simulink model "FLIGHT_hexacopter"  (R2024a)
settings: Solver=FixedStepDiscrete  StartTime=0.0  StopTime=inf  FixedStep=SampleTime_SAS  RelTol=1e-3  EnableMultiTasking=on
InitFcn:
  | Init_FLIGHT_Hexacopter
values from neighbouring files (symbols this model uses):
  d2r = pi/180    (= 0.0174532925199)    [Init_FLIGHT_Hexacopter.m]
  Kdpr = 0.004    [Init_FLIGHT_Hexacopter_fromNCMS.m]
  Kdrr = 0.004    [Init_FLIGHT_Hexacopter_fromNCMS.m]
  Kdvz = 0.0254    [Init_FLIGHT_Hexacopter_fromNCMS.m]
  Kdyr = 0.0298    [Init_FLIGHT_Hexacopter_fromNCMS.m]
  Kipr = 0.0    (= 0)    [Init_FLIGHT_Hexacopter_fromNCMS.m]
  Kirr = 0.0    (= 0)    [Init_FLIGHT_Hexacopter_fromNCMS.m]
  Kivz = 0.6304    [Init_FLIGHT_Hexacopter_fromNCMS.m]
  Kiyr = 0.0    (= 0)    [Init_FLIGHT_Hexacopter_fromNCMS.m]
  Kpp = 3.3894    [Init_FLIGHT_Hexacopter_fromNCMS.m]
  Kppr = 0.1    [Init_FLIGHT_Hexacopter_fromNCMS.m]
  Kpr = 3.3894    [Init_FLIGHT_Hexacopter_fromNCMS.m]
  Kprr = 0.1    [Init_FLIGHT_Hexacopter_fromNCMS.m]
  Kpvz = 0.3191    [Init_FLIGHT_Hexacopter_fromNCMS.m]
  Kpyr = 0.3744    [Init_FLIGHT_Hexacopter_fromNCMS.m]
  MAX_CONTROL_ANGLE_PITCH = 30*pi/180    (= 0.523598775598)    [Init_FLIGHT_Hexacopter.m]    (also in Init_FLIGHT_Hexacopter_fromNCMS.m = 0.349065850399)
  MAX_CONTROL_ANGLE_RATE_PITCH = 360*pi/180    (= 6.28318530718)    [Init_FLIGHT_Hexacopter.m]    (also in Init_FLIGHT_Hexacopter_fromNCMS.m)
  MAX_CONTROL_ANGLE_RATE_ROLL = 360*pi/180    (= 6.28318530718)    [Init_FLIGHT_Hexacopter.m]    (also in Init_FLIGHT_Hexacopter_fromNCMS.m)
  MAX_CONTROL_ANGLE_RATE_Y = 120*pi/180    (= 2.09439510239)    [Init_FLIGHT_Hexacopter.m]    (also in Init_FLIGHT_Hexacopter_fromNCMS.m)
  MAX_CONTROL_ANGLE_ROLL = 30*pi/180    (= 0.523598775598)    [Init_FLIGHT_Hexacopter.m]    (also in Init_FLIGHT_Hexacopter_fromNCMS.m = 0.349065850399)
  MAX_CONTROL_VELOCITY_XY = 1.5    [Init_FLIGHT_Hexacopter.m]    (also in Init_FLIGHT_Hexacopter_fromNCMS.m)
  MAX_CONTROL_VELOCITY_Z = 1    [Init_FLIGHT_Hexacopter.m]    (also in Init_FLIGHT_Hexacopter_fromNCMS.m)
  Npr = 50    [Init_FLIGHT_Hexacopter_fromNCMS.m]
  Nrr = 50    [Init_FLIGHT_Hexacopter_fromNCMS.m]
  Nvz = Npr    (= 50)    [Init_FLIGHT_Hexacopter_fromNCMS.m]
  Nyr = 50    [Init_FLIGHT_Hexacopter_fromNCMS.m]
  SampleTime = 1/200    (= 0.005)    [Init_FLIGHT_Hexacopter.m]    (also in Init_FLIGHT_Hexacopter_fromNCMS.m = 0.01)
  SampleTime_SAS = 1/1000    (= 0.001)    [Init_FLIGHT_Hexacopter.m]
undefined symbols (not defined in the file or in its folder): arguments, event_sequence, id, log_levels, MPC_Z_D, MPC_Z_I, MPC_Z_P, noutputs, output, pitch, pitch_body, q_d, roll, roll_body, thrust_body, timestamp, vx, vy, vz, x, y, yaw, yaw_sp_move_rate, z
libraries: px4lib x35, px4uORBlib x12, px4Utilslib x11, slpidlib x10, simulink x3, simulink_extras x2, px4Sensorslib x2, sharedtransform x1
(part 3 of 3)

== system FLIGHT_hexacopter/If Action Subsystem/XY Velocity Controller ==
  des_vxvy : Inport
  vxvy : Inport  Port=2
  Pos : Inport  Port=3
  Enable : EnablePort
  Demux : Demux  Outputs=2
  Gain1 : Gain  Gain=-1
  NED2Body1 : Subsystem
  PID_Altitude : slpidlib/PID Controller  Controller=P  Form=Parallel  TimeDomain=Discrete-time  UseExternalTs=off  SampleTime=-1  IntegratorMethod=Backward Euler  FilterMethod=Forward Euler  ControllerParametersSource=external  P=MPC_Z_P  I=MPC_Z_I  UseKiTs=off  D=MPC_Z_D  UseExternalDerivativeSource=off  N=10  UseFilter=on  TunerSelectOption=Transfer Function Based (PID Tuner App)  InitialConditionSource=internal  InitialConditionForIntegrator=0  InitialConditionForFilter=0  DifferentiatorICPrevScaledInput=0  ExternalReset=none  TrackingMode=off  Kt=1  LimitOutput=off  SatLimitsSource=internal  UpperSaturationLimit=inf  LowerSaturationLimit=-inf  LinearizeAsGain=off  AntiWindupMode=clamping  Kb=1  LimitIntegrator=off  UpperIntegratorSaturationLimit=inf  LowerIntegratorSaturationLimit=-inf  POutMin=[]  POutMax=[]  IOutMin=[]  IOutMax=[]  DOutMin=[]  DOutMax=[]  NOutMin=[]  NOutMax=[]  SumOutMin=[]  SumOutMax=[]  SaturationOutMin=[]  SaturationOutMax=[]  PParamMin=[]  PParamMax=[]  IParamMin=[]  IParamMax=[]  DParamMin=[]  DParamMax=[]  NParamMin=[]  NParamMax=[]  KbParamMin=[]  KbParamMax=[]  KtParamMin=[]  KtParamMax=[]  KbOutMin=[]  KbOutMax=[]  KtOutMin=[]  KtOutMax=[]  IntegratorOutMin=[]  IntegratorOutMax=[]  FilterOutMin=[]  FilterOutMax=[]  SumI1OutMin=[]  SumI1OutMax=[]  SumI2OutMin=[]  SumI2OutMax=[]  SumI3OutMin=[]  SumI3OutMax=[]  SumI4OutMin=[]  SumI4OutMax=[]  SumDOutMin=[]  SumDOutMax=[]  DifferentiatorOutMin=[]  DifferentiatorOutMax=[]  FilterDiffOutCoefMin=[]  FilterDiffOutCoefMax=[]  ReciprocalOutMin=[]  ReciprocalOutMax=[]  SumDenOutMin=[]  SumDenOutMax=[]  SumNumOutMin=[]  SumNumOutMax=[]  DivideOutMin=[]  DivideOutMax=[]  UdiffTsProdOutMin=[]  UdiffTsProdOutMax=[]  NTsProdOutMin=[]  NTsProdOutMax=[]  UintegralTsProdOutMin=[]  UintegralTsProdOutMax=[]  UngainTsProdOutMin=[]  UngainTsProdOutMax=[]  ClampingZeroOutDataTypeStr=Inherit: Inherit via back propagation  ClampingZeroOutMin=[]  ClampingZeroOutMax=[]  FilterDenConstantOutDataTypeStr=Inherit: Inherit via back propagation  FilterDenConstantOutMin=[]  FilterDenConstantOutMax=[]  PCopyOutDataTypeStr=Inherit: Inherit via back propagation  PCopyOutMin=[]  PCopyOutMax=[]  NCopyOutDataTypeStr=Inherit: Inherit via back propagation  NCopyOutMin=[]  NCopyOutMax=[]  IntegratorContinuousStateAttributes=''  IntegratorStateMustResolveToSignalObject=off  IntegratorRTWStateStorageClass=Auto  FilterContinuousStateAttributes=''  FilterStateMustResolveToSignalObject=off  FilterRTWStateStorageClass=Auto  ParallelPVariant=ExternalParameters  IdealPVariant=Disabled  IVariant=Disabled  DVariant=Disabled  IntegratorVariant=Disabled  SatVariant=Disabled  AWVariant=Disabled  PCopyVariant=Disabled  TRVariant=Disabled  FdbkBlocksVariant=Forward  IdealPFdbkVariant=Disabled  SatFdbkVariant=Disabled  DerivativeFilterVariant=Disabled  NVariant=Disabled  NCopyVariant=Disabled_SignalSpec  FilterICVariant=Disabled  IntegratorICVariant=Disabled  ExternalResetVariant=Disabled  TRSumVariant=Passthrough  SumFdbkVariant=Disabled  SumVariant=Passthrough_P  TsampFilterVariant=InternalTs  TsampNgainVariant=Passthrough  TsampIntegralVariant=Disabled_SignalSpec  ExternalSaturationOutDataTypeStr=Inherit: Same as second input  DerivativeSourceVariant=Disabled
  Read Parameter : px4lib/Read Parameter  ParameterName=MPC_XY_VEL_P_ACC  DataType=FLOAT  SampleTime=SampleTime
      settings: SourceProductName=UAV Toolbox Support Package for PX4 Autopilots
  Saturation : Saturate  UpperLimit=35*d2r  LowerLimit=-35*d2r
  Selector : Selector  InputPortWidth=4  IndexOptions=Index vector (dialog)  Indices=4  OutputSizes=1
  Sum : Sum  Inputs=|+-
  Terminator : Terminator
  des_pitch : Outport
  des_roll : Outport  Port=2
  wires:
  Demux/1 -> Gain1/1
  Demux/2 -> des_roll/1
  Gain1/1 -> des_pitch/1
  PID_Altitude/1 -> Saturation/1  "vz_cmd"
  Saturation/1 -> Demux/1
  Pos/1 -> Selector/1
  [heading] -> NED2Body1/2(Heading)
  des_vxvy/1 -> Sum/1
  Selector/1 -> [heading]
  vxvy/1 -> Sum/2
  Sum/1 -> NED2Body1/1(NED)
  NED2Body1/1(BODY) -> PID_Altitude/1
  Read Parameter/2 -> Terminator/1
  Read Parameter/1 -> PID_Altitude/2

== system FLIGHT_hexacopter/Remote Control/Arm1 ==
  Arm : Inport
  Compare To Constant3 : simulink/Logic and Bit Operations/Compare To Constant  relop=>=  const=uint16(1800)  OutDataTypeStr=boolean
  Arm_cmd : Outport  VectorParamsAs1DForOutWhenUnconnected=off
  wires:
  Arm/1 -> Compare To Constant3/1
  Compare To Constant3/1 -> Arm_cmd/1

== system FLIGHT_hexacopter/actuator_outputs_motors/Normalize_pwm6 ==
  In1 : Inport
  Constant : Constant  Value=1000  OutDataTypeStr=single  SampleTime=SampleTime_SAS
  Gain : Gain  Gain=1/1000
  Saturation : Saturate  UpperLimit=2000  LowerLimit=1000
  Subtract : Sum  Inputs=+-
  Out1 : Outport
  wires:
  In1/1 -> Saturation/1
  Saturation/1 -> Subtract/1
  Constant/1 -> Subtract/2
  Subtract/1 -> Gain/1
  Gain/1 -> Out1/1

== system FLIGHT_hexacopter/uORB_actuator_outputs1/Normalize_pwm6 ==
  In1 : Inport
  Constant : Constant  Value=1000  OutDataTypeStr=single
  Gain : Gain  Gain=1/1000
  Saturation : Saturate  UpperLimit=2000  LowerLimit=1000
  Subtract : Sum  Inputs=+-
  Out1 : Outport
  wires:
  In1/1 -> Saturation/1
  Saturation/1 -> Subtract/1
  Constant/1 -> Subtract/2
  Subtract/1 -> Gain/1
  Gain/1 -> Out1/1

== system FLIGHT_hexacopter/If Action Subsystem/XY Velocity Controller/NED2Body1 ==
  NED : Inport
  Heading : Inport  Port=2
  Calculate Transformation Matrix : Subsystem
  MatrixMultiply : Product  Multiplication=Matrix(*)
  BODY : Outport
  wires:
  Calculate Transformation Matrix/1(R) -> MatrixMultiply/1
  Heading/1 -> Calculate Transformation Matrix/1(theta)
  NED/1 -> MatrixMultiply/2
  MatrixMultiply/1 -> BODY/1

== system FLIGHT_hexacopter/If Action Subsystem/XY Velocity Controller/NED2Body1/Calculate Transformation Matrix ==
  theta : Inport
  Gain : Gain  Gain=-1
  Matrix Concatenate : Concatenate  Mode=Multidimensional array
  Mux : Mux  Inputs=2
  Mux1 : Mux  Inputs=2
  Reshape : Reshape  OutputDimensionality=Row vector (2-D)
  Reshape1 : Reshape  OutputDimensionality=Row vector (2-D)
  SinCos : Trigonometry  Operator=sincos
  Transpose : Math  Operator=transpose
  R : Outport
  wires:
  Reshape1/1 -> Matrix Concatenate/2
  Reshape/1 -> Matrix Concatenate/1
  Transpose/1 -> R/1
  Matrix Concatenate/1 -> Transpose/1
  Mux1/1 -> Reshape1/1
  Mux/1 -> Reshape/1
  Gain/1 -> Mux/2
  SinCos/1 -> Mux1/1, Gain/1
  SinCos/2 -> Mux/1, Mux1/2
  theta/1 -> SinCos/1

== matlab function FLIGHT_hexacopter/Doublet_Generator/MATLAB Function ==
  data: in_roll input double; in_pitch input double; in_yawrate input double; flag input boolean; out_roll output double; out_pitch output double; out_yawrate output double; time_usec input double; peak_angle_deg input double; doublet_dt input double; doublet_axis input int32
function [out_roll, out_pitch,out_yawrate]= DoubletGenerator(in_roll, in_pitch, in_yawrate, flag, time_usec, peak_angle_deg, doublet_dt, doublet_axis)
persistent start_time_usec;
if(isempty(start_time_usec))
    start_time_usec = -1;
end

if(flag && start_time_usec == -1)
    start_time_usec = time_usec;
end
d2r = pi/180;

if (flag && start_time_usec > 0) % time calculation
    reletive_time_sec = double(time_usec - start_time_usec)*1e-6;
else
    start_time_usec = -1;
    reletive_time_sec = 0;
end

% Define Doublet
t1 = 0;
t2 = t1+doublet_dt;
t3 = t2+doublet_dt;
peak_angle_rad = peak_angle_deg * d2r;

% Default Output
out_roll = in_roll;
out_pitch = in_pitch;
out_yawrate = in_yawrate;

% Generate Doublet Command
if(flag)
    if(reletive_time_sec >= t1 && reletive_time_sec < t2)
        cmd = peak_angle_rad;
    elseif(reletive_time_sec >= t2 && reletive_time_sec < t3)
        cmd = -peak_angle_rad;
    else
        cmd = 0;
    end

    switch(double(doublet_axis))
        case 1
            out_roll = cmd;
        case 2
            out_pitch = cmd;
        case 3
            out_yawrate = cmd;
    end
end

== matlab function FLIGHT_hexacopter/quat2eul ==
  data: q input; ypr output
function ypr  = quat2eul(q)

% Quaternion conversion to Euler angles based on the PX4 Firmware v1.10.2
% release.

phi = atan2(2*(q(1)*q(2) + q(3)* q(4)), q(1)^2 - q(2)^2 - q(3)^2 + q(4)^2);
theta = asin(-2*(q(2)*q(4) - q(1)*q(3)));
psi = atan2(2*(q(2)*q(3) + q(1)* q(4)), q(1)^2 + q(2)^2 - q(3)^2 - q(4)^2);

ypr = [psi theta phi];

end

== matlab function FLIGHT_hexacopter/QP_Allocation/MATLAB Function ==
  data: normalized_thrust_setpoint output size=[1 6]; f_total input; thrust_setpoints output; tau_phi input; tau_theta input; tau_psi input; A input; u_prev input double; failure_status input
function [normalized_thrust_setpoint, thrust_setpoints] = QPBasedControlAllocation(f_total, tau_phi, tau_theta, tau_psi, A, u_prev, failure_status)


% f_total: 추력 명령 [N], tau_phi, tau_theta, tau_psi: 롤 피치 요 토크 명령 [N.m]
% thrust_setpoints: 각 모터별 추력 명령[N] normalized_thrust_setpoint: 모터 최대 출력으로
% 정규화한 값
% A : Control Effectiviness MAtrix
num_actuator = 6;
u_des = [f_total; tau_phi; tau_theta; tau_psi];

% 각 추진기의 추력 제한 정의 (예시 값)
f_min = 0;           % 최소 추력 (뉴턴)
f_max = 7;           % 최대 추력 (뉴턴)

% 목적 함수의 이차 및 선형 계수 정의
% 목적: f' * f (추력의 제곱합 최소화)
H = 2 * eye(num_actuator);      % MATLAB의 quadprog은 (1/2)x'Hx + f'x를 최소화
f_obj = zeros(num_actuator,1);  % 선형 항 없음
%%
scenario = 3; 
numMotors = 6;
switch scenario
    case 1
        % 에너지 최소화: min u'u
        H = eye(numMotors);
        f_obj = zeros(numMotors,1); 
        
    case 2
        % 특정 모터 사용 억제: 모터 #1 가중치↑
        % H = diag([가중치,1,1,1,1,1])
        H = diag([1, 1, 1, 1, 1, 1]);
        f = zeros(numMotors,1);
        
    case 3
        % 추력 변화율 최소화: min (u - u_prev)'(u - u_prev)
        % = u'u - 2 u_prev'u + const
        % quadprog 형식: (1/2)*u'Hu + f'u -> 여기서 H = 2 * I, f = -2 * u_prev로 하면되지만
        % (1/2)을 빼려면 H=I로 하고 f=-2*u_prev을 그대로 써도 동일한 해를 얻기 위해,
        % 여기서는 H=I, f = -2*u_prev로 간단히 처리하겠습니다.
        
        % 실제 quadprog는 (1/2)*H*u'u + f'u를 최소화하므로
        % (1/2)*u'u + (-u_prev')*u = (1/2)*u'u - u_prev'*u
        % 이는 위 식과 상수항 차이만 있고 최소점 동일.
        H = eye(numMotors);
        f_obj = -2*u_prev; 
        % 정확히 하려면 H=2*eye(numMotors), f = -2*u_prev 로 두고,
        % 목적함수를 (1/2)*u'Hu + f'u 형태로 맞출 수 있음.
        % 여기서는 단순화해서 H=I, f=-2*u_prev 사용
        % 이 경우 목적함수는 (1/2)*u'u - u_prev'*u,
        % u'=u-u_prev일 때 상수항 무시하면 동일한 최소점.

        % 좀 더 엄밀히 하려면 다음과 같이 할 수도 있음:
        % H = 2*eye(numMotors);
        % f = -2*u_prev;
        % 이렇게 하면 목적함수는 (1/2)*u'(2I)u + (-2u_prev')u = u'u - u_prev'*u
        % = (u - u_prev)'(u - u_prev) - u_prev'u_prev (상수항 무시)
        % 이 경우가 더 직관적이므로 이렇게 하겠습니다.
        H = 2*eye(numMotors);
        f_obj = -2*u_prev;
end
%% QP
% 등식 제약 조건: A * f = u_des
Aeq = A;
beq = u_des;

failure_status = reshape(failure_status, 6, 1);

% 변수의 하한 및 상한
lb = f_min * [1 1 1 1 1 1]';
ub = f_max * failure_status;

% 이차 프로그래밍 문제 해결
options = optimoptions('quadprog', 'Display','none', 'Algorithm', 'active-set');  % 출력 숨기기
[thrust_setpoints, ~, ~, ~] = quadprog(H, f_obj, [], [], Aeq, beq, lb, ub, [0 0 0 0 0 0], options);
normalized_thrust_setpoint = thrust_setpoints ./ f_max;

== matlab function FLIGHT_hexacopter/Mixer/pwm_out2 ==
  data: Roll input; M1 output; Pitch input; Yaw input; Thrust input; M2 output; M3 output; M4 output; M5 output; M6 output
function [M1, M2, M3, M4, M5, M6] = motor_mixer(Roll, Pitch, Yaw, Thrust)
%Function description:
%  Control allocation. The quadrotor type is X-configuration,
%  and the airframe is as follows:
%3↓   1↑
 %  \ /
 %  / \
 %2↑   4↓
%Input：
%  Roll, Pitch, Yaw: attitude controller output.
%  Thrust

idle_PWM = 1000;
scale = 1000;
scale_att = scale*Thrust;

% M1 = uint16(Thrust*scale + (- Roll + Pitch + Yaw) * scale_att + idle_PWM);
% M2 = uint16(Thrust*scale + (Roll - Pitch + Yaw) * scale_att + idle_PWM);
% M3 = uint16(Thrust*scale + (Roll + Pitch - Yaw) * scale_att + idle_PWM);
% M4 = uint16(Thrust*scale + (- Roll - Pitch - Yaw) * scale_att + idle_PWM);

% Hex X
% M1 = ((Pitch + Roll / 2 - Yaw) * Thrust / 2 + Thrust) * 1000 + idle_PWM;
% M2 = ((Pitch - Roll / 2 + Yaw) * Thrust / 2 + Thrust) * 1000 + idle_PWM;
% M3 = ((-Roll - Yaw) * Thrust / 2 + Thrust) * 1000 + idle_PWM;
% M4 = ((-Pitch - Roll / 2 + Yaw) * Thrust / 2 + Thrust) * 1000 + idle_PWM;
% M5 = ((-Pitch + Roll / 2 - Yaw) * Thrust / 2 + Thrust) * 1000 + idle_PWM;
% M6 = ((Roll + Yaw) * Thrust / 2 + Thrust) * 1000 + idle_PWM;
% M7 = 1000;
% M8 = 1000;

% Hex X (From Adam)
M1 = uint16(single(((-Roll - Yaw) * Thrust / 3 + Thrust) * single(1000))) + idle_PWM;
M2 = uint16(single(((Roll + Yaw) * Thrust / 3 + Thrust) * single(1000))) + idle_PWM;
M3 = uint16(single(((Pitch + (Roll / 2) - Yaw) * Thrust / 3 + Thrust) * single(1000))) + idle_PWM;
M4 = uint16(single(((-Pitch - (Roll / 2) + Yaw) * Thrust / 3 + Thrust) * single(1000))) + idle_PWM;
M5 = uint16(single(((Pitch - (Roll / 2) + Yaw) * Thrust / 3 + Thrust) * single(1000))) + idle_PWM;
M6 = uint16(single(((-Pitch + (Roll / 2) - Yaw) * Thrust / 3 + Thrust) * single(1000))) + idle_PWM;

% Hex X (Version 2)
% Roll/Yaw
% M1 = ((-Roll - Yaw) * Thrust / 2 + Thrust) * 1000 + idle_PWM;
% M2 = ((Roll + Yaw) * Thrust / 2 + Thrust) * 1000 + idle_PWM;
% % + Pitch/Roll
% M6 = ((Pitch + Roll / 2 - Yaw) * Thrust / 2 + Thrust) * 1000 + idle_PWM;
% M4 = ((Pitch - Roll / 2 + Yaw) * Thrust / 2 + Thrust) * 1000 + idle_PWM;
% % - Pitch/Roll
% M5 = ((-Pitch - Roll / 2 + Yaw) * Thrust / 2 + Thrust) * 1000 + idle_PWM;
% M3 = ((-Pitch + Roll / 2 - Yaw) * Thrust / 2 + Thrust) * 1000 + idle_PWM;
